simulink model "greenhouse_simulink_part_1_2"  (R2023b)
settings: Solver=VariableStepAuto  StartTime=0.0  StopTime=60*60*24  RelTol=1e-3
undefined symbols (not defined in the file or in its folder): Ca, km1_m2, km1e, km2e, p, t0, Ts
settings Model: Creator=bianc  LastModifiedBy=bianc
settings OptimizationCC: ReuseModelBlockBuffer=off

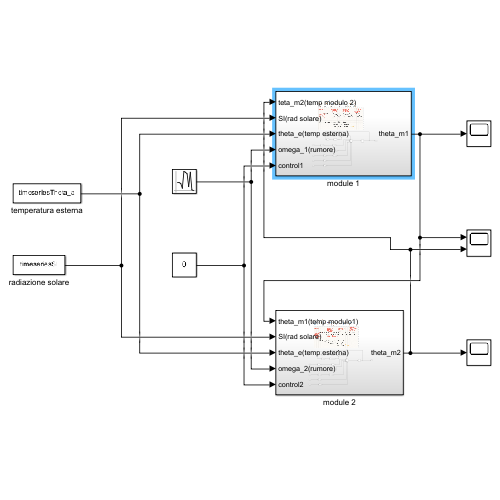
[thumbnail: Simulink's stored preview of the top-level diagram]
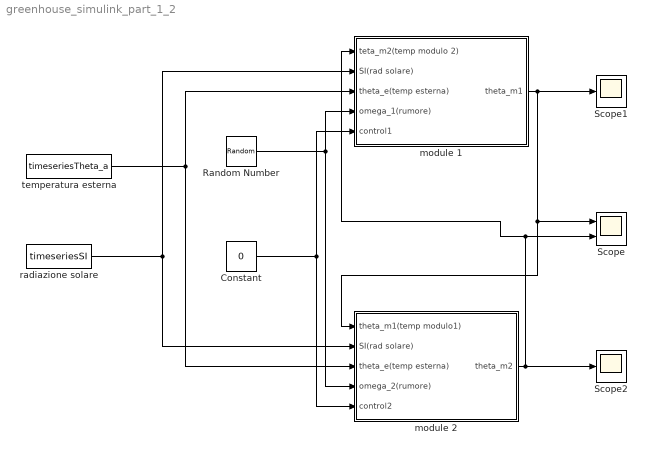
== system greenhouse_simulink_part_1_2 ==
  Constant : Constant  Value=0
  Random Number : RandomNumber  SampleTime=1
  Scope : Scope  NumInputPorts=2
  Scope1 : Scope
  Scope2 : Scope
  module 1 : Subsystem
  module 2 : Subsystem
  radiazione solare : FromWorkspace  VariableName=timeseriesSI
  temperatura esterna : FromWorkspace  VariableName=timeseriesTheta_a
  wires:
  radiazione solare/1 -> module 2/2(SI(rad solare)), module 1/2(SI(rad solare))
  temperatura esterna/1 -> module 2/3(theta_e(temp esterna)), module 1/3(theta_e(temp esterna))
  Random Number/1 -> module 2/4(omega_2(rumore)), module 1/4(omega_1(rumore))
  Constant/1 -> module 2/5(control2), module 1/5(control1)
  module 1/1(theta_m1) -> Scope1/1, module 2/1(theta_m1(temp modulo1)), Scope/1
  module 2/1(theta_m2) -> Scope2/1, module 1/1(teta_m2(temp modulo 2)), Scope/2

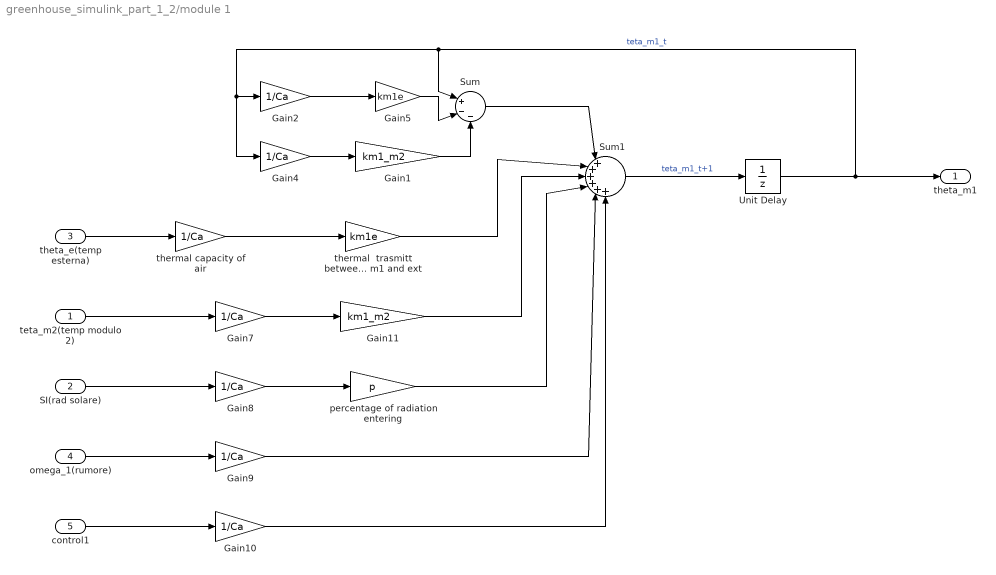
== system greenhouse_simulink_part_1_2/module 1 ==
  teta_m2(temp modulo 2) : Inport
  SI(rad solare) : Inport  Port=2
  theta_e(temp esterna) : Inport  Port=3
  omega_1(rumore) : Inport  Port=4
  control1 : Inport  Port=5
  Gain1 : Gain  Gain=km1_m2
  Gain{2,4,7..10} (6 alike) : Gain  Gain=1/Ca
  Gain11 : Gain  Gain=km1_m2
  Gain5 : Gain  Gain=km1e
  Sum : Sum  Inputs=|+--
  Sum1 : Sum  Inputs=|++++++
  Unit Delay : UnitDelay  InitialCondition=t0  SampleTime=Ts  HasFrameUpgradeWarning=on
  percentage of radiation entering : Gain  Gain=p
  thermal  trasmitt between air in m1 and ext : Gain  Gain=km1e
  thermal capacity of air : Gain  Gain=1/Ca
  theta_m1 : Outport
  wires:
  Unit Delay/1 -> Gain4/1, Gain2/1, Sum/1, theta_m1/1  "teta_m1_t"
  control1/1 -> Gain10/1
  Sum/1 -> Sum1/1
  teta_m2(temp modulo 2)/1 -> Gain7/1
  omega_1(rumore)/1 -> Gain9/1
  thermal  trasmitt between air in m1 and ext/1 -> Sum1/2
  Sum1/1 -> Unit Delay/1  "teta_m1_t+1"
  Gain11/1 -> Sum1/3
  percentage of radiation entering/1 -> Sum1/4
  SI(rad solare)/1 -> Gain8/1
  theta_e(temp esterna)/1 -> thermal capacity of air/1
  Gain2/1 -> Gain5/1
  Gain4/1 -> Gain1/1
  thermal capacity of air/1 -> thermal  trasmitt between air in m1 and ext/1
  Gain7/1 -> Gain11/1
  Gain8/1 -> percentage of radiation entering/1
  Gain9/1 -> Sum1/5
  Gain10/1 -> Sum1/6
  Gain5/1 -> Sum/2
  Gain1/1 -> Sum/3

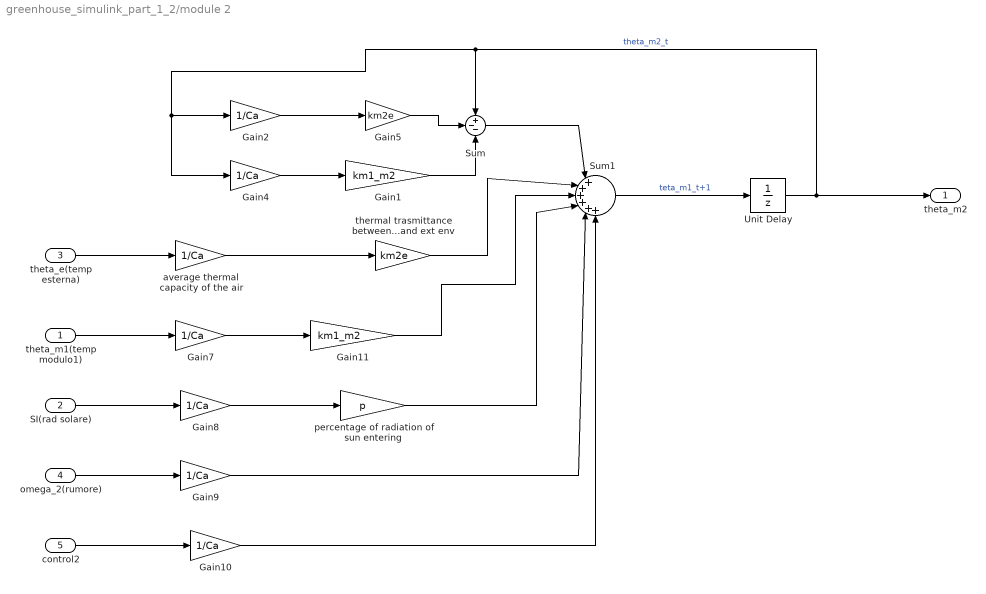
== system greenhouse_simulink_part_1_2/module 2 ==
  theta_m1(temp modulo1) : Inport
  SI(rad solare) : Inport  Port=2
  theta_e(temp esterna) : Inport  Port=3
  omega_2(rumore) : Inport  Port=4
  control2 : Inport  Port=5
  Gain1 : Gain  Gain=km1_m2
  Gain{2,4,7..10} (6 alike) : Gain  Gain=1/Ca
  Gain11 : Gain  Gain=km1_m2
  Gain5 : Gain  Gain=km2e
  Sum : Sum  Inputs=+--
  Sum1 : Sum  Inputs=|++++++
  Unit Delay : UnitDelay  InitialCondition=t0  SampleTime=Ts  HasFrameUpgradeWarning=on
  average thermal capacity of the air : Gain  Gain=1/Ca
  percentage of radiation of sun entering : Gain  Gain=p
  thermal trasmittance between module 2 and ext env : Gain  Gain=km2e
  theta_m2 : Outport
  wires:
  Unit Delay/1 -> Sum/1, Gain4/1, Gain2/1, theta_m2/1  "theta_m2_t"
  control2/1 -> Gain10/1
  Sum/1 -> Sum1/1
  theta_m1(temp modulo1)/1 -> Gain7/1
  omega_2(rumore)/1 -> Gain9/1
  thermal trasmittance between module 2 and ext env/1 -> Sum1/2
  Gain11/1 -> Sum1/3
  percentage of radiation of sun entering/1 -> Sum1/4
  SI(rad solare)/1 -> Gain8/1
  theta_e(temp esterna)/1 -> average thermal capacity of the air/1
  Gain2/1 -> Gain5/1
  Gain4/1 -> Gain1/1
  average thermal capacity of the air/1 -> thermal trasmittance between module 2 and ext env/1
  Gain7/1 -> Gain11/1
  Gain8/1 -> percentage of radiation of sun entering/1
  Gain9/1 -> Sum1/5
  Gain10/1 -> Sum1/6
  Sum1/1 -> Unit Delay/1  "teta_m1_t+1"
  Gain5/1 -> Sum/2
  Gain1/1 -> Sum/3
